simulink model "APPModeDetector"  (R2022b)
settings: Solver=FixedStepDiscrete  StartTime=0.0  StopTime=10.0  FixedStep=0.1  RelTol=1e-3
undefined symbols (not defined in the file or in its folder): APP_Modes
settings Model: Creator=ahmed  LastModifiedBy=ahmed

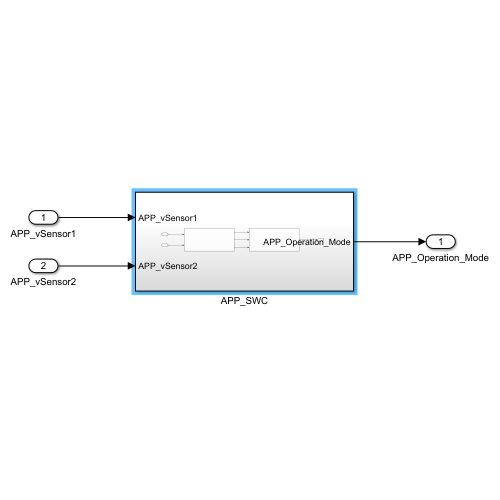
[thumbnail: Simulink's stored preview of the top-level diagram]
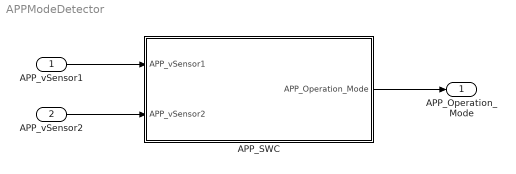
== system APPModeDetector ==
  APP_vSensor1 : Inport  OutDataTypeStr=single
  APP_vSensor2 : Inport  Port=2  OutDataTypeStr=single
  APP_SWC : Subsystem
  APP_Operation_Mode : Outport  OutDataTypeStr=Enum: APP_Modes
  wires:
  APP_vSensor1/1 -> APP_SWC/1(APP_vSensor1)
  APP_vSensor2/1 -> APP_SWC/2(APP_vSensor2)
  APP_SWC/1(APP_Operation_Mode) -> APP_Operation_Mode/1

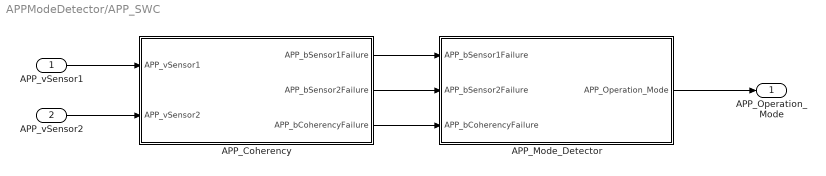
== system APPModeDetector/APP_SWC ==
  APP_vSensor1 : Inport  OutDataTypeStr=single
  APP_vSensor2 : Inport  Port=2  OutDataTypeStr=single
  APP_Coherency : Subsystem
  APP_Mode_Detector : Subsystem
  APP_Operation_Mode : Outport  OutDataTypeStr=Enum: APP_Modes
  wires:
  APP_vSensor2/1 -> APP_Coherency/2(APP_vSensor2)
  APP_Coherency/3(APP_bCoherencyFailure) -> APP_Mode_Detector/3(APP_bCoherencyFailure)
  APP_Mode_Detector/1(APP_Operation_Mode) -> APP_Operation_Mode/1
  APP_Coherency/1(APP_bSensor1Failure) -> APP_Mode_Detector/1(APP_bSensor1Failure)
  APP_vSensor1/1 -> APP_Coherency/1(APP_vSensor1)
  APP_Coherency/2(APP_bSensor2Failure) -> APP_Mode_Detector/2(APP_bSensor2Failure)

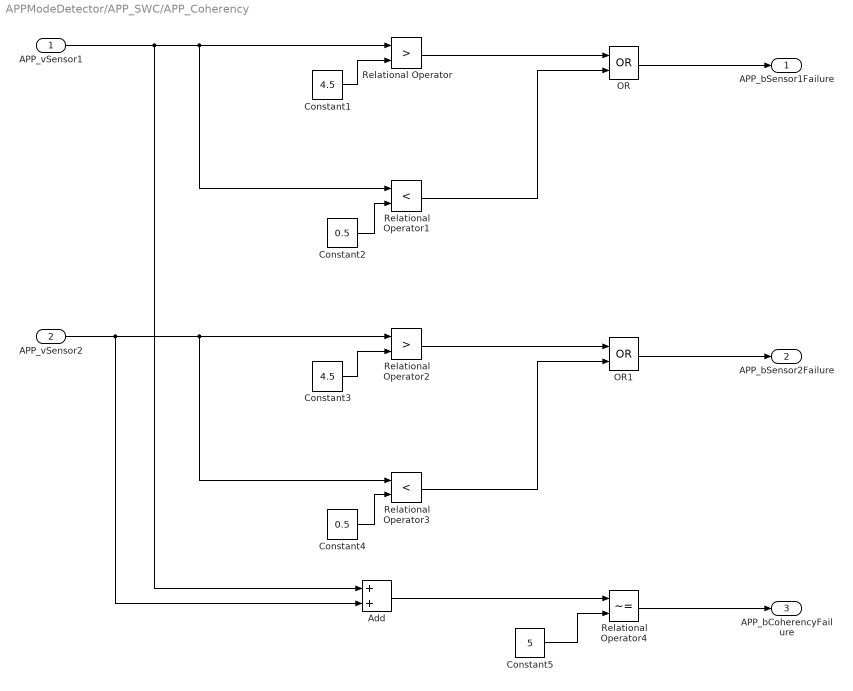
== system APPModeDetector/APP_SWC/APP_Coherency ==
  APP_vSensor1 : Inport  OutDataTypeStr=single
  APP_vSensor2 : Inport  Port=2  OutDataTypeStr=single
  Add : Sum
  Constant1 : Constant  Value=4.5
  Constant2 : Constant  Value=0.5
  Constant3 : Constant  Value=4.5
  Constant4 : Constant  Value=0.5
  Constant5 : Constant  Value=5
  OR : Logic  Operator=OR  AllPortsSameDT=off  OutDataTypeStr=boolean
  OR1 : Logic  Operator=OR  AllPortsSameDT=off  OutDataTypeStr=boolean
  Relational Operator : RelationalOperator  Operator=>  OutDataTypeStr=boolean  RndMeth=Simplest  InputSameDT=off
  Relational Operator1 : RelationalOperator  Operator=<  OutDataTypeStr=boolean  RndMeth=Simplest  InputSameDT=off
  Relational Operator2 : RelationalOperator  Operator=>  OutDataTypeStr=boolean  RndMeth=Simplest  InputSameDT=off
  Relational Operator3 : RelationalOperator  Operator=<  OutDataTypeStr=boolean  RndMeth=Simplest  InputSameDT=off
  Relational Operator4 : RelationalOperator  Operator=~=  OutDataTypeStr=boolean  RndMeth=Simplest  InputSameDT=off
  APP_bSensor1Failure : Outport  OutDataTypeStr=boolean
  APP_bSensor2Failure : Outport  Port=2  OutDataTypeStr=boolean
  APP_bCoherencyFailure : Outport  Port=3  OutDataTypeStr=boolean
  wires:
  Relational Operator4/1 -> APP_bCoherencyFailure/1
  APP_vSensor1/1 -> Relational Operator1/1, Relational Operator/1, Add/1
  Constant5/1 -> Relational Operator4/2
  OR/1 -> APP_bSensor1Failure/1
  Relational Operator1/1 -> OR/2
  Constant4/1 -> Relational Operator3/2
  Constant1/1 -> Relational Operator/2
  OR1/1 -> APP_bSensor2Failure/1
  Constant2/1 -> Relational Operator1/2
  Add/1 -> Relational Operator4/1
  Relational Operator2/1 -> OR1/1
  Relational Operator/1 -> OR/1
  APP_vSensor2/1 -> Relational Operator3/1, Relational Operator2/1, Add/2
  Constant3/1 -> Relational Operator2/2
  Relational Operator3/1 -> OR1/2

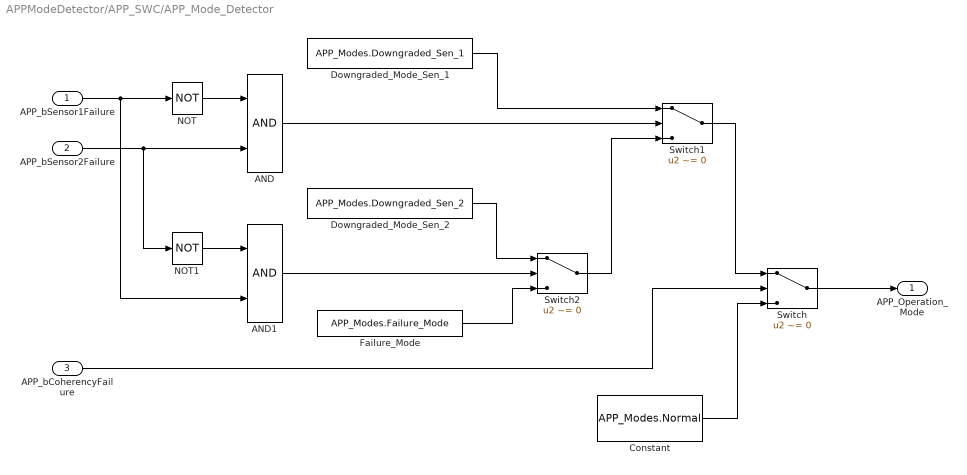
== system APPModeDetector/APP_SWC/APP_Mode_Detector ==
  APP_bSensor1Failure : Inport  OutDataTypeStr=boolean
  APP_bSensor2Failure : Inport  Port=2  OutDataTypeStr=boolean
  APP_bCoherencyFailure : Inport  Port=3  OutDataTypeStr=boolean
  AND : Logic  AllPortsSameDT=off  OutDataTypeStr=boolean
  AND1 : Logic  AllPortsSameDT=off  OutDataTypeStr=boolean
  Constant : Constant  Value=APP_Modes.Normal
  Downgraded_Mode_Sen_1 : Constant  Value=APP_Modes.Downgraded_Sen_1
  Downgraded_Mode_Sen_2 : Constant  Value=APP_Modes.Downgraded_Sen_2
  Failure_Mode : Constant  Value=APP_Modes.Failure_Mode
  NOT : Logic  Operator=NOT  AllPortsSameDT=off  OutDataTypeStr=boolean
  NOT1 : Logic  Operator=NOT  AllPortsSameDT=off  OutDataTypeStr=boolean
  Switch : Switch  Criteria=u2 ~= 0  SaturateOnIntegerOverflow=off  InputSameDT=off
  Switch1 : Switch  Criteria=u2 ~= 0  SaturateOnIntegerOverflow=off  InputSameDT=off
  Switch2 : Switch  Criteria=u2 ~= 0  SaturateOnIntegerOverflow=off  InputSameDT=off
  APP_Operation_Mode : Outport  OutDataTypeStr=Enum: APP_Modes
  wires:
  APP_bCoherencyFailure/1 -> Switch/2
  Constant/1 -> Switch/3
  APP_bSensor1Failure/1 -> NOT/1, AND1/2
  NOT/1 -> AND/1
  APP_bSensor2Failure/1 -> AND/2, NOT1/1
  AND/1 -> Switch1/2
  Downgraded_Mode_Sen_1/1 -> Switch1/1
  NOT1/1 -> AND1/1
  Downgraded_Mode_Sen_2/1 -> Switch2/1
  AND1/1 -> Switch2/2
  Failure_Mode/1 -> Switch2/3
  Switch2/1 -> Switch1/3
  Switch1/1 -> Switch/1
  Switch/1 -> APP_Operation_Mode/1
